simulink subsystem "SiEngine"  (R2023a)
settings: Solver=VariableStepAuto  StartTime=0.0  StopTime=10.0  RelTol=1e-3
undefined symbols (not defined in the file): PlntEngAfrStoich, PlntEngTimeCECP, PlntEngTimeCEGR, PlntEngTimeCETC, PlntEngTimeCICP, PlntEngTimeCIRL, PlntEngTimeCIVL, PlntEngTimeCVCR, PlntEngTimeCVGT, PlntEngTimeCWGA, PlntEngTimeCWVA, PlntEngTwcEffCO, PlntEngTwcEffHC, PlntEngTwcEffLam, PlntEngTwcEffNOx
libraries: autolibhevctrlrcommon x1, autolibpowerinfoutils x1, autolibutils x1
settings Model: ModifiedByFormat=The MathWorks, Inc.  Creator=The MathWorks, Inc.  LastModifiedBy=The MathWorks, Inc.
settings SolverCC: MaxZcPerStep=1
settings DebuggingCC: UnconnectedInputMsg=warning  UnconnectedOutputMsg=warning  UnconnectedLineMsg=warning
settings ModelReferenceCC: EnableRefExpFcnMdlSchedulingChecks=on
settings RTWCC: DLArmComputeVersion=19.05

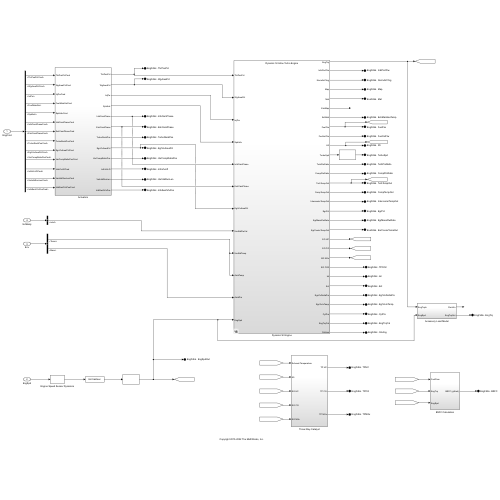
[thumbnail: Simulink's stored preview of the top-level diagram]
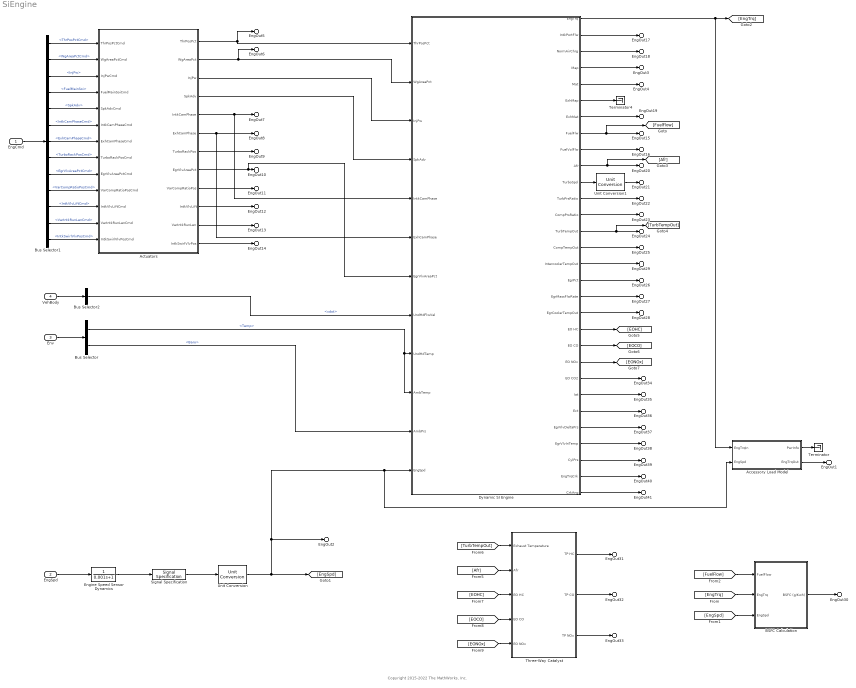
== system SiEngine ==
  note: Copyright 2015-2022 The MathWorks, Inc.
  EngCmd : Inport
  EngSpd : Inport  Port=2  Unit=rad/sec
  Env : Inport  Port=3
  VehBody : Inport  Port=4
  Accessory Load Model : Subsystem
  Actuators : Subsystem
  BSFC Calculation : Subsystem
  Bus Selector : BusSelector  OutputSignals=Temp,Baro
  Bus Selector1 : BusSelector  OutputSignals=ThrPosPctCmd,WgAreaPctCmd,InjPw,FuelMainSoi,SpkAdv,IntkCamPhaseCmd,ExhCamPhaseCmd,TurboRackPosCmd,EgrVlvAreaPctCmd,VarCompRatioPosCmd,IntkVlvLiftCmd,VarIntkRunLenCmd,IntkSwirlVlvPosCmd
  Bus Selector2 : BusSelector  OutputSignals=BdyFrm.Cg.Vel.xdot
  Dynamic SI Engine : Subsystem  Variant=on  VariantControlMode=label  VariantControl=Choice  LabelModeActiveChoice=SiEngineCore
  Engine Speed Sensor Dynamics : TransferFcn  Denominator=[0.001 1]
  Signal Specification : SignalSpecification  Unit=rad/sec
  Terminator : Terminator
  Terminator4 : Terminator
  Three-Way Catalyst : Subsystem
  Unit Conversion : UnitConversion
  Unit Conversion1 : UnitConversion
  EngOut1 : Outport  PortName=EngFdbk  Element=EngTrq
  EngOut2 : Outport  PortName=EngFdbk  Element=EngSpdOut
  EngOut3 : Outport  PortName=EngFdbk  Element=Map
  EngOut4 : Outport  PortName=EngFdbk  Element=Mat
  EngOut5 : Outport  PortName=EngFdbk  Element=ThrPosPct
  EngOut6 : Outport  PortName=EngFdbk  Element=WgAreaPct
  EngOut7 : Outport  PortName=EngFdbk  Element=IntkCamPhase
  EngOut8 : Outport  PortName=EngFdbk  Element=ExhCamPhase
  EngOut9 : Outport  PortName=EngFdbk  Element=TurboRackPos
  EngOut10 : Outport  PortName=EngFdbk  Element=EgrVlvAreaPct
  EngOut11 : Outport  PortName=EngFdbk  Element=VarCompRatioPos
  EngOut12 : Outport  PortName=EngFdbk  Element=IntkVlvLift
  EngOut13 : Outport  PortName=EngFdbk  Element=VarIntkRunLen
  EngOut14 : Outport  PortName=EngFdbk  Element=IntkSwirlVlvPos
  EngOut15 : Outport  PortName=EngFdbk  Element=FuelFlw
  EngOut16 : Outport  PortName=EngFdbk  Element=FuelVolFlw
  EngOut17 : Outport  PortName=EngFdbk  Element=IntkPortFlw
  EngOut18 : Outport  PortName=EngFdbk  Element=NormAirChrg
  EngOut19 : Outport  PortName=EngFdbk  Element=ExhManGasTemp
  EngOut20 : Outport  PortName=EngFdbk  Element=Afr
  EngOut21 : Outport  PortName=EngFdbk  Element=TurboSpd
  EngOut22 : Outport  PortName=EngFdbk  Element=TurbPrsRatio
  EngOut23 : Outport  PortName=EngFdbk  Element=CompPrsRatio
  EngOut24 : Outport  PortName=EngFdbk  Element=TurbTempOut
  EngOut25 : Outport  PortName=EngFdbk  Element=CompTempOut
  EngOut26 : Outport  PortName=EngFdbk  Element=EgrPct
  EngOut27 : Outport  PortName=EngFdbk  Element=EgrMassFlwRate
  EngOut28 : Outport  PortName=EngFdbk  Element=EgrCoolerTempOut
  EngOut29 : Outport  PortName=EngFdbk  Element=IntercoolerTempOut
  EngOut30 : Outport  PortName=EngFdbk  Element=BSFC
  EngOut31 : Outport  PortName=EngFdbk  Element=TPHC
  EngOut32 : Outport  PortName=EngFdbk  Element=TPCO
  EngOut33 : Outport  PortName=EngFdbk  Element=TPNOx
  EngOut34 : Outport  PortName=EngFdbk  Element=TPCO2
  EngOut35 : Outport  PortName=EngFdbk  Element=Iat
  EngOut36 : Outport  PortName=EngFdbk  Element=Ect
  EngOut37 : Outport  PortName=EngFdbk  Element=EgrVlvDeltaPrs
  EngOut38 : Outport  PortName=EngFdbk  Element=EgrVlvInTemp
  EngOut39 : Outport  PortName=EngFdbk  Element=CylPrs
  EngOut40 : Outport  PortName=EngFdbk  Element=EngTrqCrk
  EngOut41 : Outport  PortName=EngFdbk  Element=CrkAng
  wires:
  Engine Speed Sensor Dynamics/1 -> Signal Specification/1
  VehBody/1 -> Bus Selector2/1
  Env/1 -> Bus Selector/1
  Unit Conversion/1 -> Dynamic SI Engine/12(EngSpd), Accessory Load Model/2(EngSpd), EngOut2/1, [EngSpd]
  Dynamic SI Engine/29(EngTrqCrk) -> EngOut40/1
  Dynamic SI Engine/18(EgrMassFlwRate) -> EngOut27/1
  Dynamic SI Engine/30(CrkAng) -> EngOut41/1
  Dynamic SI Engine/28(CylPrs) -> EngOut39/1
  Dynamic SI Engine/27(EgrVlvInTemp) -> EngOut38/1
  Actuators/9(VarCompRatioPos) -> EngOut11/1
  Dynamic SI Engine/24(Iat) -> EngOut35/1
  Dynamic SI Engine/21(EO CO) -> [EOCO]
  Accessory Load Model/2(EngTrqOut) -> EngOut1/1
  Actuators/6(ExhCamPhase) -> EngOut8/1, Dynamic SI Engine/6(ExhCamPhase)
  Actuators/1(ThrPosPct) -> EngOut5/1, Dynamic SI Engine/1(ThrPosPct)
  Dynamic SI Engine/4(Map) -> EngOut3/1
  Accessory Load Model/1(PwrInfo) -> Terminator/1
  Dynamic SI Engine/26(EgrVlvDeltaPrs) -> EngOut37/1
  Actuators/2(WgAreaPct) -> EngOut6/1, Dynamic SI Engine/2(WgAreaPct)
  Dynamic SI Engine/25(Ect) -> EngOut36/1
  Dynamic SI Engine/16(IntercoolerTempOut) -> EngOut29/1
  Dynamic SI Engine/7(ExhMat) -> EngOut19/1
  BSFC Calculation/1(BSFC (g/Kwh)) -> EngOut30/1
  Dynamic SI Engine/23(EO CO2) -> EngOut34/1
  Actuators/7(TurboRackPos) -> EngOut9/1
  Dynamic SI Engine/15(CompTempOut) -> EngOut25/1
  Dynamic SI Engine/14(TurbTempOut) -> EngOut24/1, [TurbTempOut]
  Dynamic SI Engine/22(EO NOx) -> [EONOx]
  Actuators/10(IntkVlvLift) -> EngOut12/1
  Dynamic SI Engine/1(EngTrq) -> [EngTrq], Accessory Load Model/1(EngTrqIn)
  Dynamic SI Engine/13(CompPrsRatio) -> EngOut23/1
  Dynamic SI Engine/20(EO HC) -> [EOHC]
  Actuators/8(EgrVlvAreaPct) -> EngOut10/1, Dynamic SI Engine/7(EgrVlvAreaPct)
  Dynamic SI Engine/5(Mat) -> EngOut4/1
  Actuators/3(InjPw) -> Dynamic SI Engine/3(InjPw)
  Dynamic SI Engine/2(IntkPortFlw) -> EngOut17/1
  [EONOx] -> Three-Way Catalyst/5(EO NOx)
  Bus Selector/1 -> Dynamic SI Engine/9(UndHdTemp), Dynamic SI Engine/10(AmbTemp)  "<Temp>"
  Actuators/4(SpkAdv) -> Dynamic SI Engine/4(SpkAdv)
  Dynamic SI Engine/9(FuelVolFlw) -> EngOut16/1
  Dynamic SI Engine/19(EgrCoolerTempOut) -> EngOut28/1
  Actuators/12(IntkSwirlVlvPos) -> EngOut14/1
  EngSpd/1 -> Engine Speed Sensor Dynamics/1
  Dynamic SI Engine/3(NormAirChrg) -> EngOut18/1
  Bus Selector2/1 -> Dynamic SI Engine/8(UndHdFlwVel)  "<xdot>"
  [EOHC] -> Three-Way Catalyst/3(EO HC)
  [EngTrq] -> BSFC Calculation/2(EngTrq)
  Actuators/5(IntkCamPhase) -> EngOut7/1, Dynamic SI Engine/5(IntkCamPhase)
  [Afr] -> Three-Way Catalyst/2(Afr)
  Three-Way Catalyst/2(TP CO) -> EngOut32/1
  [EngSpd] -> BSFC Calculation/3(EngSpd)
  Dynamic SI Engine/12(TurbPrsRatio) -> EngOut22/1
  Bus Selector/2 -> Dynamic SI Engine/11(AmbPrs)  "<Baro>"
  [FuelFlow] -> BSFC Calculation/1(FuelFlow)
  Dynamic SI Engine/17(EgrPct) -> EngOut26/1
  Three-Way Catalyst/3(TP NOx) -> EngOut33/1
  Dynamic SI Engine/6(ExhMap) -> Terminator4/1
  [EOCO] -> Three-Way Catalyst/4(EO CO)
  Actuators/11(VarIntkRunLen) -> EngOut13/1
  Three-Way Catalyst/1(TP HC) -> EngOut31/1
  [TurbTempOut] -> Three-Way Catalyst/1(Exhaust Temperature)
  Dynamic SI Engine/8(FuelFlw) -> [FuelFlow], EngOut15/1
  Dynamic SI Engine/10(Afr) -> [Afr], EngOut20/1
  EngCmd/1 -> Bus Selector1/1
  Bus Selector1/5 -> Actuators/5(SpkAdvCmd)  "<SpkAdv>"
  Bus Selector1/9 -> Actuators/9(EgrVlvAreaPctCmd)  "<EgrVlvAreaPctCmd>"
  Bus Selector1/11 -> Actuators/11(IntkVlvLiftCmd)  "<IntkVlvLiftCmd>"
  Bus Selector1/13 -> Actuators/13(IntkSwirlVlvPosCmd)  "<IntkSwirlVlvPosCmd>"
  Bus Selector1/8 -> Actuators/8(TurboRackPosCmd)  "<TurboRackPosCmd>"
  Bus Selector1/4 -> Actuators/4(FuelMainSoiCmd)  "<FuelMainSoi>"
  Bus Selector1/12 -> Actuators/12(VarIntkRunLenCmd)  "<VarIntkRunLenCmd>"
  Bus Selector1/2 -> Actuators/2(WgAreaPctCmd)  "<WgAreaPctCmd>"
  Bus Selector1/3 -> Actuators/3(InjPwCmd)  "<InjPw>"
  Bus Selector1/6 -> Actuators/6(IntkCamPhaseCmd)  "<IntkCamPhaseCmd>"
  Bus Selector1/10 -> Actuators/10(VarCompRatioPosCmd)  "<VarCompRatioPosCmd>"
  Bus Selector1/1 -> Actuators/1(ThrPosPctCmd)  "<ThrPosPctCmd>"
  Bus Selector1/7 -> Actuators/7(ExhCamPhaseCmd)  "<ExhCamPhaseCmd>"
  Dynamic SI Engine/11(TurboSpd) -> Unit Conversion1/1
  Unit Conversion1/1 -> EngOut21/1
  Signal Specification/1 -> Unit Conversion/1

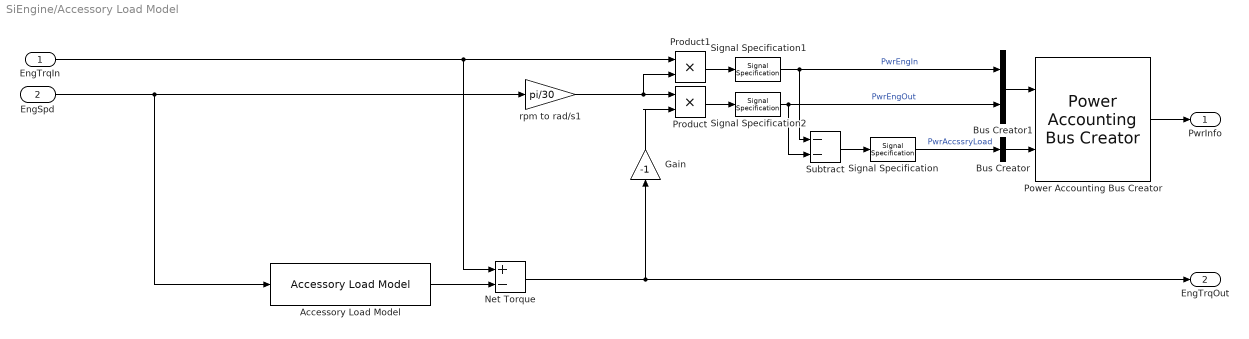
== system SiEngine/Accessory Load Model ==
  EngTrqIn : Inport
  EngSpd : Inport  Port=2
  Accessory Load Model : autolibhevctrlrcommon/Accessory Load Model  AccPwrTbl=PlntEngAccPwrTbl  AccSpdBpts=PlntEngAccSpdBpt
  Bus Creator : BusCreator  Inputs=1
  Bus Creator1 : BusCreator  Inputs=2
  Gain : Gain  Gain=-1
  Net Torque : Sum  Inputs=+-
  Power Accounting Bus Creator : autolibpowerinfoutils/Power Accounting Bus Creator  AssctBlkSelPopup=Parent  RefBlkName='libraryname/blkname'  PwrTrnsfrdCheckBox=on  PwrNotTrnsfrdCheckBox=on  PwrStoredCheckBox=off  aMode=aMode
  Product : Product
  Product1 : Product
  Signal Specification : SignalSpecification  Unit=W
  Signal Specification1 : SignalSpecification  Unit=W
  Signal Specification2 : SignalSpecification  Unit=W
  Subtract : Sum  Inputs=--
  rpm to rad/s1 : Gain  Gain=pi/30
  PwrInfo : Outport  VectorParamsAs1DForOutWhenUnconnected=off
  EngTrqOut : Outport  Port=2  Unit=N*m  VectorParamsAs1DForOutWhenUnconnected=off
  wires:
  Accessory Load Model/1 -> Net Torque/2
  EngSpd/1 -> Accessory Load Model/1, rpm to rad/s1/1
  Net Torque/1 -> EngTrqOut/1, Gain/1
  Bus Creator/1 -> Power Accounting Bus Creator/2
  Bus Creator1/1 -> Power Accounting Bus Creator/1
  EngTrqIn/1 -> Product1/1, Net Torque/1
  Subtract/1 -> Signal Specification/1
  Signal Specification/1 -> Bus Creator/1  "PwrAccssryLoad"
  Power Accounting Bus Creator/1 -> PwrInfo/1
  Product/1 -> Signal Specification2/1
  Product1/1 -> Signal Specification1/1
  rpm to rad/s1/1 -> Product1/2, Product/1
  Signal Specification1/1 -> Subtract/1, Bus Creator1/1  "PwrEngIn"
  Signal Specification2/1 -> Subtract/2, Bus Creator1/2  "PwrEngOut"
  Gain/1 -> Product/2

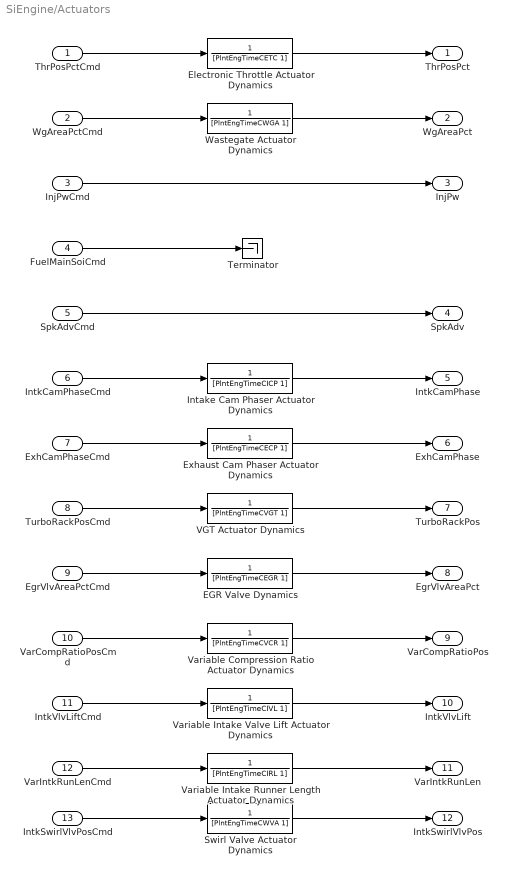
== system SiEngine/Actuators ==
  ThrPosPctCmd : Inport  Unit=%
  WgAreaPctCmd : Inport  Port=2  Unit=%
  InjPwCmd : Inport  Port=3  Unit=ms
  FuelMainSoiCmd : Inport  Port=4  Unit=deg
  SpkAdvCmd : Inport  Port=5  Unit=deg
  IntkCamPhaseCmd : Inport  Port=6  Unit=deg
  ExhCamPhaseCmd : Inport  Port=7  Unit=deg
  TurboRackPosCmd : Inport  Port=8  Unit=1
  EgrVlvAreaPctCmd : Inport  Port=9  Unit=%
  VarCompRatioPosCmd : Inport  Port=10
  IntkVlvLiftCmd : Inport  Port=11
  VarIntkRunLenCmd : Inport  Port=12
  IntkSwirlVlvPosCmd : Inport  Port=13
  EGR Valve Dynamics : TransferFcn  Denominator=[PlntEngTimeCEGR 1]
  Electronic Throttle Actuator Dynamics : TransferFcn  Denominator=[PlntEngTimeCETC 1]
  Exhaust Cam Phaser Actuator Dynamics : TransferFcn  Denominator=[PlntEngTimeCECP 1]
  Intake Cam Phaser Actuator Dynamics : TransferFcn  Denominator=[PlntEngTimeCICP 1]
  Swirl Valve Actuator Dynamics : TransferFcn  Denominator=[PlntEngTimeCWVA 1]
  Terminator : Terminator
  VGT Actuator Dynamics : TransferFcn  Denominator=[PlntEngTimeCVGT 1]
  Variable Compression Ratio Actuator Dynamics : TransferFcn  Denominator=[PlntEngTimeCVCR 1]
  Variable Intake Runner Length Actuator Dynamics : TransferFcn  Denominator=[PlntEngTimeCIRL 1]
  Variable Intake Valve Lift Actuator Dynamics : TransferFcn  Denominator=[PlntEngTimeCIVL 1]
  Wastegate Actuator Dynamics : TransferFcn  Denominator=[PlntEngTimeCWGA 1]
  ThrPosPct : Outport  Unit=%  VectorParamsAs1DForOutWhenUnconnected=off
  WgAreaPct : Outport  Port=2  Unit=%  VectorParamsAs1DForOutWhenUnconnected=off
  InjPw : Outport  Port=3  VectorParamsAs1DForOutWhenUnconnected=off
  SpkAdv : Outport  Port=4  VectorParamsAs1DForOutWhenUnconnected=off
  IntkCamPhase : Outport  Port=5  Unit=deg  VectorParamsAs1DForOutWhenUnconnected=off
  ExhCamPhase : Outport  Port=6  Unit=deg  VectorParamsAs1DForOutWhenUnconnected=off
  TurboRackPos : Outport  Port=7  Unit=1  VectorParamsAs1DForOutWhenUnconnected=off
  EgrVlvAreaPct : Outport  Port=8  Unit=%  VectorParamsAs1DForOutWhenUnconnected=off
  VarCompRatioPos : Outport  Port=9  VectorParamsAs1DForOutWhenUnconnected=off
  IntkVlvLift : Outport  Port=10  VectorParamsAs1DForOutWhenUnconnected=off
  VarIntkRunLen : Outport  Port=11  VectorParamsAs1DForOutWhenUnconnected=off
  IntkSwirlVlvPos : Outport  Port=12  VectorParamsAs1DForOutWhenUnconnected=off
  wires:
  Variable Compression Ratio Actuator Dynamics/1 -> VarCompRatioPos/1
  Variable Intake Valve Lift Actuator Dynamics/1 -> IntkVlvLift/1
  Variable Intake Runner Length Actuator Dynamics/1 -> VarIntkRunLen/1
  Swirl Valve Actuator Dynamics/1 -> IntkSwirlVlvPos/1
  Intake Cam Phaser Actuator Dynamics/1 -> IntkCamPhase/1
  Exhaust Cam Phaser Actuator Dynamics/1 -> ExhCamPhase/1
  Wastegate Actuator Dynamics/1 -> WgAreaPct/1
  Electronic Throttle Actuator Dynamics/1 -> ThrPosPct/1
  FuelMainSoiCmd/1 -> Terminator/1
  IntkVlvLiftCmd/1 -> Variable Intake Valve Lift Actuator Dynamics/1
  IntkSwirlVlvPosCmd/1 -> Swirl Valve Actuator Dynamics/1
  WgAreaPctCmd/1 -> Wastegate Actuator Dynamics/1
  ThrPosPctCmd/1 -> Electronic Throttle Actuator Dynamics/1
  ExhCamPhaseCmd/1 -> Exhaust Cam Phaser Actuator Dynamics/1
  IntkCamPhaseCmd/1 -> Intake Cam Phaser Actuator Dynamics/1
  VarCompRatioPosCmd/1 -> Variable Compression Ratio Actuator Dynamics/1
  VarIntkRunLenCmd/1 -> Variable Intake Runner Length Actuator Dynamics/1
  InjPwCmd/1 -> InjPw/1
  VGT Actuator Dynamics/1 -> TurboRackPos/1
  EGR Valve Dynamics/1 -> EgrVlvAreaPct/1
  TurboRackPosCmd/1 -> VGT Actuator Dynamics/1
  EgrVlvAreaPctCmd/1 -> EGR Valve Dynamics/1
  SpkAdvCmd/1 -> SpkAdv/1

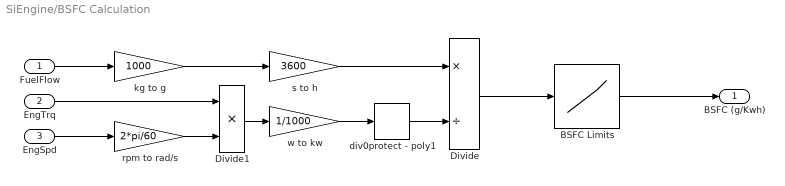
== system SiEngine/BSFC Calculation ==
  FuelFlow : Inport
  EngTrq : Inport  Port=2
  EngSpd : Inport  Port=3
  BSFC Limits : Lookup_n-D  NumberOfTableDimensions=1  BreakpointsForDimension1=[0 500]  Table=[0 500]  ExtrapMethod=Clip  InternalRulePriority=Speed  RndMeth=Simplest
  Divide : Product  Inputs=*/
  Divide1 : Product  Inputs=**
  div0protect - poly1 : autolibutils/div0protect - poly  thresh=1e-6  ZeroCross1=off  aMode=aMode
  kg to g : Gain  Gain=1000
  rpm to rad/s : Gain  Gain=2*pi/60
  s to h : Gain  Gain=3600
  w to kw : Gain  Gain=1/1000
  BSFC (g/Kwh) : Outport  VectorParamsAs1DForOutWhenUnconnected=off
  wires:
  Divide1/1 -> w to kw/1
  kg to g/1 -> s to h/1
  FuelFlow/1 -> kg to g/1
  rpm to rad/s/1 -> Divide1/2
  EngSpd/1 -> rpm to rad/s/1
  EngTrq/1 -> Divide1/1
  Divide/1 -> BSFC Limits/1
  w to kw/1 -> div0protect - poly1/1
  s to h/1 -> Divide/1
  BSFC Limits/1 -> BSFC (g/Kwh)/1
  div0protect - poly1/1 -> Divide/2

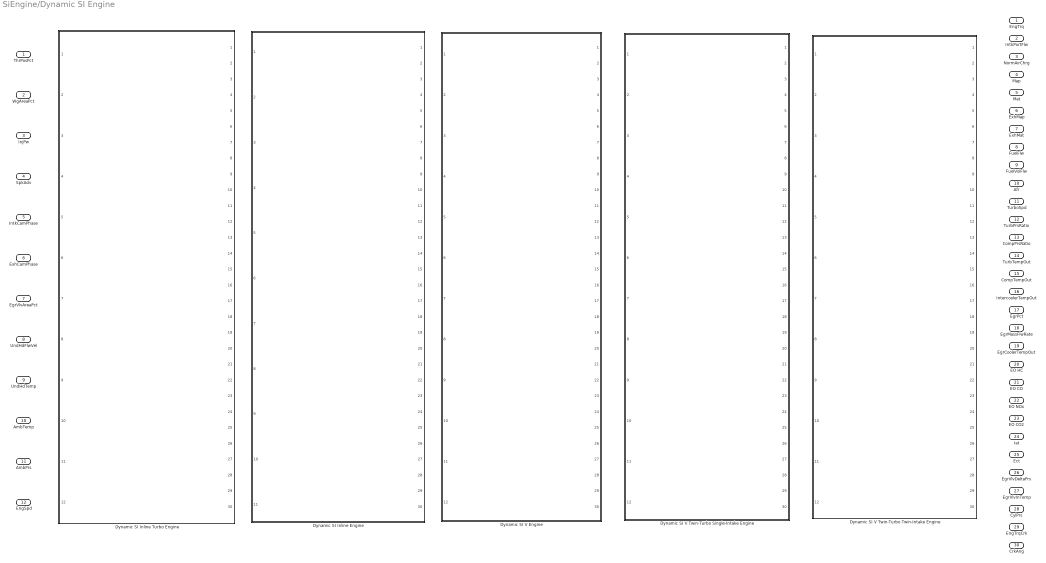
== system SiEngine/Dynamic SI Engine ==
  ThrPosPct : Inport
  WgAreaPct : Inport  Port=2
  InjPw : Inport  Port=3
  SpkAdv : Inport  Port=4
  IntkCamPhase : Inport  Port=5
  ExhCamPhase : Inport  Port=6
  EgrVlvAreaPct : Inport  Port=7
  UndHdFlwVel : Inport  Port=8
  UndHdTemp : Inport  Port=9
  AmbTemp : Inport  Port=10
  AmbPrs : Inport  Port=11
  EngSpd : Inport  Port=12
  Dynamic SI Inline Engine : Subsystem  VariantControl=SiEngineCoreNA  ReferencedSubsystem=SiEngineCoreNA
  Dynamic SI Inline Turbo Engine : Subsystem  VariantControl=SiEngineCore  ReferencedSubsystem=SiEngineCore
  Dynamic SI V Engine : Subsystem  VariantControl=SiEngineCoreVNA  ReferencedSubsystem=SiEngineCoreVNA
  Dynamic SI V Twin-Turbo Single-Intake Engine : Subsystem  VariantControl=SiEngineCoreV  ReferencedSubsystem=SiEngineCoreV
  Dynamic SI V Twin-Turbo Twin-Intake Engine : Subsystem  VariantControl=SiEngineCoreVThr2  ReferencedSubsystem=SiEngineCoreVThr2
  EngTrq : Outport
  IntkPortFlw : Outport  Port=2
  NormAirChrg : Outport  Port=3
  Map : Outport  Port=4
  Mat : Outport  Port=5
  ExhMap : Outport  Port=6
  ExhMat : Outport  Port=7
  FuelFlw : Outport  Port=8
  FuelVolFlw : Outport  Port=9
  Afr : Outport  Port=10
  TurboSpd : Outport  Port=11
  TurbPrsRatio : Outport  Port=12
  CompPrsRatio : Outport  Port=13
  TurbTempOut : Outport  Port=14
  CompTempOut : Outport  Port=15
  IntercoolerTempOut : Outport  Port=16
  EgrPct : Outport  Port=17
  EgrMassFlwRate : Outport  Port=18
  EgrCoolerTempOut : Outport  Port=19
  EO HC : Outport  Port=20
  EO CO : Outport  Port=21
  EO NOx : Outport  Port=22
  EO CO2 : Outport  Port=23
  Iat : Outport  Port=24
  Ect : Outport  Port=25
  EgrVlvDeltaPrs : Outport  Port=26
  EgrVlvInTemp : Outport  Port=27
  CylPrs : Outport  Port=28  VectorParamsAs1DForOutWhenUnconnected=off
  EngTrqCrk : Outport  Port=29  VectorParamsAs1DForOutWhenUnconnected=off
  CrkAng : Outport  Port=30  VectorParamsAs1DForOutWhenUnconnected=off

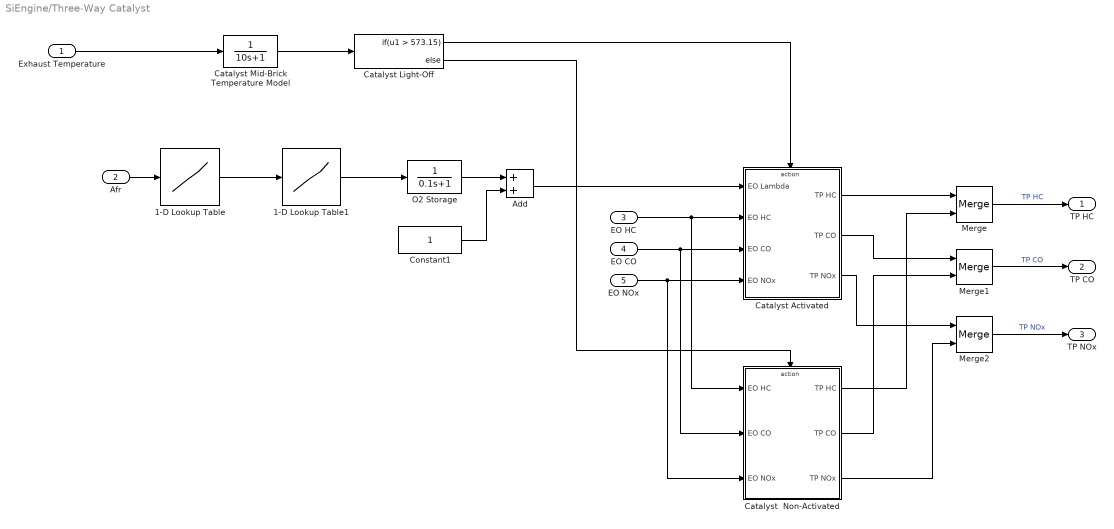
== system SiEngine/Three-Way Catalyst ==
  Exhaust Temperature : Inport
  Afr : Inport  Port=2
  EO HC : Inport  Port=3
  EO CO : Inport  Port=4
  EO NOx : Inport  Port=5
  1-D Lookup Table : Lookup_n-D  NumberOfTableDimensions=1  BreakpointsForDimension1=[0 15 100]  Table=[0 15 PlntEngAfrStoich]/PlntEngAfrStoich  ExtrapMethod=Clip  InternalRulePriority=Speed  RndMeth=Simplest
  1-D Lookup Table1 : Lookup_n-D  NumberOfTableDimensions=1  BreakpointsForDimension1=[0 0.97 1.03 1.1]  Table=[-1 0 0 0.07]  ExtrapMethod=Clip  InternalRulePriority=Speed  RndMeth=Simplest
  Add : Sum
  Catalyst  Non-Activated : Subsystem
  Catalyst Activated : Subsystem
  Catalyst Light-Off : If  IfExpression=u1 > 573.15
  "Catalyst Mid-Brick Temperature Model " : TransferFcn  Denominator=[10 1]
  Constant1 : Constant
  Merge : Merge
  Merge1 : Merge
  Merge2 : Merge
  O2 Storage : TransferFcn  Denominator=[0.1 1]
  TP HC : Outport  Unit=kg/s  VectorParamsAs1DForOutWhenUnconnected=off
  TP CO : Outport  Port=2  Unit=kg/s  VectorParamsAs1DForOutWhenUnconnected=off
  TP NOx : Outport  Port=3  Unit=kg/s  VectorParamsAs1DForOutWhenUnconnected=off
  wires:
  EO HC/1 -> Catalyst  Non-Activated/1(EO HC), Catalyst Activated/2(EO HC)
  EO CO/1 -> Catalyst  Non-Activated/2(EO CO), Catalyst Activated/3(EO CO)
  EO NOx/1 -> Catalyst  Non-Activated/3(EO NOx), Catalyst Activated/4(EO NOx)
  Merge/1 -> TP HC/1  "TP HC"
  Merge1/1 -> TP CO/1  "TP CO"
  Merge2/1 -> TP NOx/1  "TP NOx"
  Exhaust Temperature/1 -> "Catalyst Mid-Brick Temperature Model "/1
  Catalyst Light-Off/1 -> Catalyst Activated/Action
  Catalyst Light-Off/2 -> Catalyst  Non-Activated/Action
  "Catalyst Mid-Brick Temperature Model "/1 -> Catalyst Light-Off/1
  Catalyst Activated/1(TP HC) -> Merge/1
  Catalyst  Non-Activated/1(TP HC) -> Merge/2
  Catalyst Activated/2(TP CO) -> Merge1/1
  Catalyst  Non-Activated/2(TP CO) -> Merge1/2
  Catalyst Activated/3(TP NOx) -> Merge2/1
  Catalyst  Non-Activated/3(TP NOx) -> Merge2/2
  Add/1 -> Catalyst Activated/1(EO Lambda)
  1-D Lookup Table1/1 -> O2 Storage/1
  Constant1/1 -> Add/2
  O2 Storage/1 -> Add/1
  Afr/1 -> 1-D Lookup Table/1
  1-D Lookup Table/1 -> 1-D Lookup Table1/1

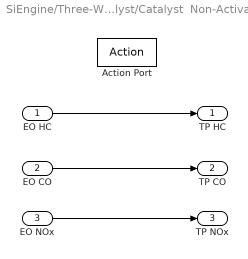
== system SiEngine/Three-Way Catalyst/Catalyst  Non-Activated ==
  EO HC : Inport
  EO CO : Inport  Port=2
  EO NOx : Inport  Port=3
  Action Port : ActionPort
  TP HC : Outport  VectorParamsAs1DForOutWhenUnconnected=off
  TP CO : Outport  Port=2  VectorParamsAs1DForOutWhenUnconnected=off
  TP NOx : Outport  Port=3  VectorParamsAs1DForOutWhenUnconnected=off
  wires:
  EO HC/1 -> TP HC/1
  EO CO/1 -> TP CO/1
  EO NOx/1 -> TP NOx/1

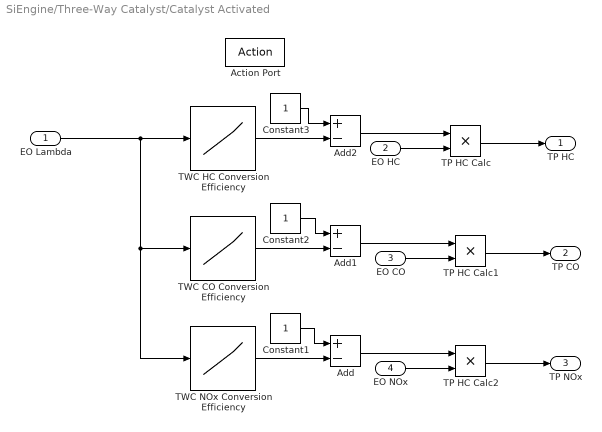
== system SiEngine/Three-Way Catalyst/Catalyst Activated ==
  EO Lambda : Inport
  EO HC : Inport  Port=2
  EO CO : Inport  Port=3
  EO NOx : Inport  Port=4
  Action Port : ActionPort
  Add : Sum  Inputs=+-
  Add1 : Sum  Inputs=+-
  Add2 : Sum  Inputs=+-
  Constant1 : Constant
  Constant2 : Constant
  Constant3 : Constant
  TP HC Calc : Product  Inputs=**
  TP HC Calc1 : Product  Inputs=**
  TP HC Calc2 : Product  Inputs=**
  TWC CO Conversion Efficiency : Lookup_n-D  NumberOfTableDimensions=1  LookupTableObject=''  BreakpointsForDimension1=PlntEngTwcEffLam  Table=PlntEngTwcEffCO  ExtrapMethod=Clip  InternalRulePriority=Speed  RndMeth=Simplest
  TWC HC Conversion Efficiency : Lookup_n-D  NumberOfTableDimensions=1  LookupTableObject=''  BreakpointsForDimension1=PlntEngTwcEffLam  Table=PlntEngTwcEffHC  ExtrapMethod=Clip  InternalRulePriority=Speed  RndMeth=Simplest
  TWC NOx Conversion Efficiency : Lookup_n-D  NumberOfTableDimensions=1  LookupTableObject=''  BreakpointsForDimension1=PlntEngTwcEffLam  Table=PlntEngTwcEffNOx  ExtrapMethod=Clip  InternalRulePriority=Speed  RndMeth=Simplest
  TP HC : Outport  VectorParamsAs1DForOutWhenUnconnected=off
  TP CO : Outport  Port=2  VectorParamsAs1DForOutWhenUnconnected=off
  TP NOx : Outport  Port=3  VectorParamsAs1DForOutWhenUnconnected=off
  wires:
  EO HC/1 -> TP HC Calc/2
  TP HC Calc/1 -> TP HC/1
  Add/1 -> TP HC Calc2/1
  Constant1/1 -> Add/1
  TP HC Calc1/1 -> TP CO/1
  TWC HC Conversion Efficiency/1 -> Add2/2
  Add1/1 -> TP HC Calc1/1
  EO CO/1 -> TP HC Calc1/2
  TP HC Calc2/1 -> TP NOx/1
  EO NOx/1 -> TP HC Calc2/2
  EO Lambda/1 -> TWC NOx Conversion Efficiency/1, TWC CO Conversion Efficiency/1, TWC HC Conversion Efficiency/1
  Constant2/1 -> Add1/1
  TWC CO Conversion Efficiency/1 -> Add1/2
  Constant3/1 -> Add2/1
  Add2/1 -> TP HC Calc/1
  TWC NOx Conversion Efficiency/1 -> Add/2
